simulink model "Adaptive_Fuzzy_HVS"  (R2024b)
settings: Solver=ode4  StartTime=0.0  StopTime=120  FixedStep=0.01  MaxStep=0.01  MinStep=1e-6  RelTol=1e-4  AbsTol=1e-6
values from neighbouring files (symbols this model uses):
  eta_0 = [-0.04; 3.52; 3.45; 0; 0; -1.87]    [Init_AUV_Params.m]    (also in main.m)
  M_inv = inv(M_mat)    [Init_AUV_Params.m]    (also in controller_fuzzy.m = inv(diag([98+49, 98+49, 98+49, 8, 8, 8])); main.m)
  nu_0 = zeros(6,1)    [Init_AUV_Params.m]    (also in main.m)
  q_j = -4 + 8 * rand(18, num_rules)    [Init_AUV_Params.m]
  s1_0 = 6.75    [Init_AUV_Params.m]    (also in main.m)
  xi_hat = [120; 160; 27; 0; 0; -1.87]    [Init_AUV_Params.m]    (also in Run_Monte_Carlo.m = evalin('base', 'xi_hat'); main.m)
settings Model: Creator=Alany  LastModifiedBy=Alany

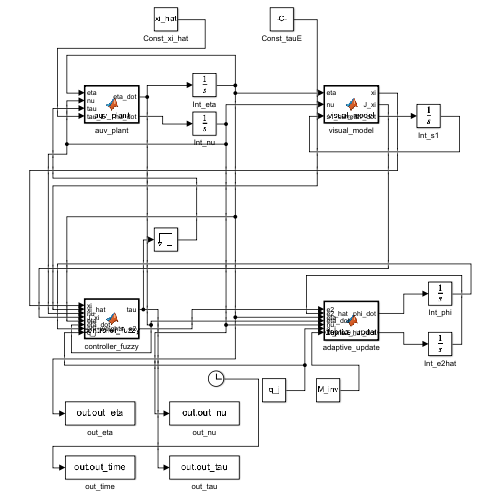
[thumbnail: Simulink's stored preview of the top-level diagram]
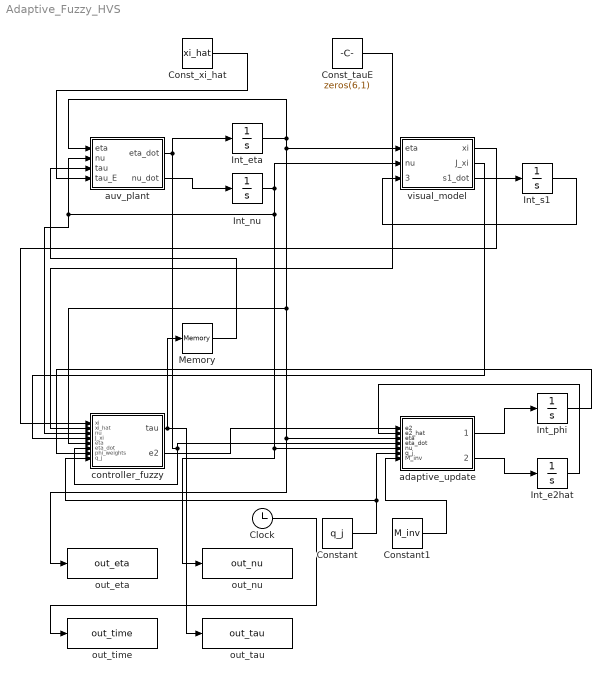
== system Adaptive_Fuzzy_HVS ==
  Clock : Clock
  Const_tauE : Constant  Value=zeros(6,1)
  Const_xi_hat : Constant  Value=xi_hat
  Constant : Constant  Value=q_j
  Constant1 : Constant  Value=M_inv
  Int_e2hat : Integrator  InitialCondition=zeros(6,1)
  Int_eta : Integrator  InitialCondition=eta_0
  Int_nu : Integrator  InitialCondition=nu_0
  Int_phi : Integrator  InitialCondition=zeros(17,6)
  Int_s1 : Integrator  InitialCondition=s1_0
  Memory : Memory  InitialCondition=zeros(6,1)
  adaptive_update : MATLAB Function  TreatAsAtomicUnit=on
  auv_plant : MATLAB Function  TreatAsAtomicUnit=on
  controller_fuzzy : MATLAB Function  TreatAsAtomicUnit=on
  out_eta : ToWorkspace  VariableName=out_eta  SampleTime=-1
  out_nu : ToWorkspace  VariableName=out_nu  SampleTime=-1
  out_tau : ToWorkspace  VariableName=out_tau  SampleTime=-1
  out_time : ToWorkspace  VariableName=out_time  SampleTime=-1
  visual_model : MATLAB Function  TreatAsAtomicUnit=on
  wires:
  auv_plant/2(nu_dot) -> Int_nu/1
  adaptive_update/1(phi_dot) -> Int_phi/1
  adaptive_update/2(e2_hat_dot) -> Int_e2hat/1
  Int_s1/1 -> visual_model/3(s1_current)
  Int_eta/1 -> out_eta/1, adaptive_update/3(eta), controller_fuzzy/5(eta), visual_model/1(eta), auv_plant/1(eta)
  Int_nu/1 -> visual_model/2(nu), out_nu/1, adaptive_update/5(nu), controller_fuzzy/3(nu), auv_plant/2(nu)
  Int_phi/1 -> controller_fuzzy/7(phi_weights)
  Int_e2hat/1 -> adaptive_update/2(e2_hat)
  controller_fuzzy/2(e2) -> adaptive_update/1(e2)
  controller_fuzzy/1(tau) -> Memory/1, out_tau/1
  Const_tauE/1 -> controller_fuzzy/2(xi_hat)
  Const_xi_hat/1 -> auv_plant/4(tau_E)
  visual_model/1(xi) -> controller_fuzzy/1(xi)
  visual_model/2(J_xi) -> controller_fuzzy/4(J_xi)
  Clock/1 -> out_time/1
  visual_model/3(s1_dot) -> Int_s1/1
  auv_plant/1(eta_dot) -> Int_eta/1, adaptive_update/4(eta_dot), controller_fuzzy/6(eta_dot)
  Memory/1 -> auv_plant/3(tau)
  Constant/1 -> adaptive_update/6(q_j), controller_fuzzy/8(q_j)
  Constant1/1 -> adaptive_update/7(M_inv)

== matlab function Adaptive_Fuzzy_HVS/visual_model ==
  data: eta input; xi output; nu input; s1_current input; J_xi output; s1_dot output
function [xi, J_xi, s1_dot] = visual_model(eta, nu, s1_current)
    % 修复：基于论文 Eq(3) 与 Eq(11) 补全真实的相机相对投影关系
    
    % 提取状态
    x = eta(1); y = eta(2); z = eta(3);
    phi = eta(4); theta = eta(5); psi = eta(6);
    Z_depth = abs(z) + 0.01; % 深度防除零
    
    % --- 关键修复：反推的虚拟相机内参与目标全局坐标 ---
    % 论文稳态 AUV 位姿为 [1.9, 4.5, 0.5]，稳态视觉特征为 [120, 160]
    % 假设目标固定在海底 P_target = [3.4, 6.5, 0] (满足投影关系)
    f_x = 40; f_y = 40; 
    c_x = 0; c_y = 0;
    
    X_rel = 3.4 - x; 
    Y_rel = 6.5 - y;
    
    % 计算像素平面的投影特征
    x_v = f_y * X_rel / Z_depth + c_y; 
    x_u = f_x * Y_rel / Z_depth + c_x;
    
    xi = [x_v; x_u; s1_current; phi; theta; psi];
    
    % 计算图像雅可比矩阵 J_xi
    a1 = x_v - c_y; 
    a2 = x_u - c_x;
    L_R_Z = [-f_y/Z_depth,  0,             a1/Z_depth,  a1*a2/f_x,                  -(f_y^2+a1^2)/f_y, a2*f_y/f_x;
              0,            -f_x/Z_depth,  a2/Z_depth,  (f_x^2+a2^2)/f_x,           -a1*a2/f_y,        -a1*f_x/f_y];
    
    J3 = [-sin(theta), cos(theta)*sin(phi), cos(theta)*cos(phi)];
    J2 = [1, sin(phi)*tan(theta), cos(phi)*tan(theta);
          0, cos(phi),           -sin(phi);
          0, sin(phi)/cos(theta), cos(phi)/cos(theta)];
    
    J_xi = [L_R_Z;
            (2*s1_current/Z_depth)*J3, zeros(1,3);
            zeros(3,3), J2];
            
    % 面积特征动态方程 Eq(5)
    Z_dot = -J3 * nu(1:3); 
    s1_dot = (-2 * s1_current / Z_depth) * Z_dot;
end

== matlab function Adaptive_Fuzzy_HVS/auv_plant ==
  data: eta input; eta_dot output; nu input; tau input; tau_E input; nu_dot output
function [eta_dot, nu_dot] = auv_plant(eta, nu, tau, tau_E)
    % 提取从工作区加载的全局参数
    m = 98.0; W = 961.38; B = 952.56; x_G = 0; y_G = 0; z_G = 0.05;
    X_u_dot = 49.0; Y_v_dot = 49.0; Z_w_dot = 49.0; I_x = 8.0; I_y = 8.0; I_z = 8.0;
    X_uu = -148.0; Y_vv = -148.0; Z_ww = -148.0; K_pp = -180.0; M_qq = -180.0; N_rr = -180.0;
    K_p = -130.0; M_q = -130.0; N_r = -130.0;
    
    phi = eta(4); theta = eta(5); psi = eta(6);
    u = nu(1); v = nu(2); w = nu(3); p = nu(4); q = nu(5); r = nu(6);
    
    % 运动学矩阵
    J1 = [cos(psi)*cos(theta), -sin(psi)*cos(phi)+cos(psi)*sin(theta)*sin(phi),  sin(psi)*sin(phi)+cos(psi)*cos(phi)*sin(theta);
          sin(psi)*cos(theta),  cos(psi)*cos(phi)+sin(phi)*sin(theta)*sin(psi), -cos(psi)*sin(phi)+sin(theta)*sin(psi)*cos(phi);
         -sin(theta),         cos(theta)*sin(phi),                            cos(theta)*cos(phi)];
    J2 = [1, sin(phi)*tan(theta), cos(phi)*tan(theta);
          0, cos(phi),           -sin(phi);
          0, sin(phi)/cos(theta), cos(phi)/cos(theta)];
    J_eta = blkdiag(J1, J2);
    eta_dot = J_eta * nu;
    
    % 动力学矩阵
    M = diag([m+X_u_dot, m+Y_v_dot, m+Z_w_dot, I_x, I_y, I_z]);
    D = -diag([X_uu*abs(u), Y_vv*abs(v), Z_ww*abs(w), K_p+K_pp*abs(p), M_q+M_qq*abs(q), N_r+N_rr*abs(r)]);
    
    % 简化的向心力矩阵 C
    C = zeros(6,6);
    C(1,5) = M(3,3)*w; C(1,6) = -M(2,2)*v;
    C(2,4) = -M(3,3)*w; C(2,6) = M(1,1)*u;
    C(3,4) = M(2,2)*v; C(3,5) = -M(1,1)*u;
    C(4,5) = -M(6,6)*r; C(4,6) = M(5,5)*q;
    C(5,4) = M(6,6)*r; C(5,6) = -M(4,4)*p;
    C(6,4) = -M(5,5)*q; C(6,5) = M(4,4)*p;
    C = C - C';
    
    % 恢复力与力矩 g
    g = [(W-B)*sin(theta);
         -(W-B)*cos(theta)*sin(phi);
         -(W-B)*cos(theta)*cos(phi);
         y_G*W*cos(theta)*cos(phi) - z_G*W*cos(theta)*sin(phi);
         -x_G*W*cos(theta)*cos(phi) - z_G*W*sin(theta);
         x_G*W*cos(theta)*sin(phi) + y_G*W*sin(theta)];
    
    % 求解加速度
    nu_dot = M \ (tau + tau_E - C*nu - D*nu - g);
end

== matlab function Adaptive_Fuzzy_HVS/controller_fuzzy ==
  data: xi input; tau output; xi_hat input; nu input; J_xi input; eta input; eta_dot input; phi_weights input; e2 output; q_j input
function [tau, e2] = controller_fuzzy(xi, xi_hat, nu, J_xi, eta, eta_dot, phi_weights, q_j)
    % 1. 强制定义输出维度，规避编译报错
    tau = zeros(6, 1);
    e2 = zeros(6, 1);

    % 2. 内部控制参数
    k1 = 2; 
    k2 = 100; 
    d_j = 2;
    
    % 3. 虚拟控制律与误差计算
    e1 = xi - xi_hat;
    alpha_1 = -pinv(J_xi) * (k1 * e1);
    e2 = nu - alpha_1;

    % 4. 模糊逻辑系统基函数 (q_j 现在从外部信号线传进来，完美绕过编译限制)
    gamma = [eta; eta_dot; nu];
    S_gamma_unnorm = zeros(17, 1);
    for i = 1:17
        S_gamma_unnorm(i) = exp(-norm(gamma - q_j(:,i))^2 / d_j^2);
    end
    S_gamma = S_gamma_unnorm / (sum(S_gamma_unnorm) + 1e-6);

    % 5. 实际控制指令 (推力)
    tau = phi_weights' * S_gamma - k2 * e2;
end

== matlab function Adaptive_Fuzzy_HVS/adaptive_update ==
  data: e2 input; phi_dot output; e2_hat input; eta input; eta_dot input; nu input; e2_hat_dot output; q_j input; M_inv input
function [phi_dot, e2_hat_dot] = adaptive_update(e2, e2_hat, eta, eta_dot, nu, q_j, M_inv)
    % 1. 强制定义输出维度
    phi_dot = zeros(17, 6);
    e2_hat_dot = zeros(6, 1);

    % 2. 内部控制参数
    k2 = 100; 
    d_j = 2;
    b1 = 50 * eye(6);
    k3 = diag([90, 90, 5, 1, 1, 1]);

    % 3. 指令滤波器
    e2_hat_dot = -b1 * (e2_hat - e2);

    % 4. 重新计算高斯基底 (q_j 从外部传入)
    gamma = [eta; eta_dot; nu];
    S_gamma_unnorm = zeros(17, 1);
    for i = 1:17
        S_gamma_unnorm(i) = exp(-norm(gamma - q_j(:,i))^2 / d_j^2);
    end
    S_gamma = S_gamma_unnorm / (sum(S_gamma_unnorm) + 1e-6);

    % 5. 计算权重导数 (M_inv 从外部传入)
    for i = 1:6
        phi_dot(:, i) = k3(i,i) * (e2_hat_dot(i) + k2 * M_inv(i,i) * e2(i)) * S_gamma;
    end
end
